simulink model "mini_projekt"  (R2020a)
settings: Solver=VariableStepAuto  StartTime=0.0  StopTime=10.0  MaxStep=0.1  RelTol=1e-3
values from neighbouring files (symbols this model uses):
  cp = 1000    [Skrypt.m]    (also in proj.m)
  Cv1 = cp*rop*V1    (= 90000)    [Skrypt.m]    (also in proj.m)
  Cv2 = cp*rop*V2    (= 90000)    [Skrypt.m]    (also in proj.m)
  dfp0 = 0*fpN    (= 0)    [Skrypt.m]    (also in proj.m)
  dTkz0 = 0    [Skrypt.m]    (also in proj.m)
  dTzew0 = 0    [Skrypt.m]    (also in proj.m)
  fp0 = fpN    (= 1.66666666667)    [Skrypt.m]    (also in proj.m)
  K0 = (qkN - Ks1*(Tw1N-TzewN))/(Tw1N-Tw2N)    (= 1600)    [Skrypt.m]    (also in proj.m)
  Ks1 = 0.6*qkN/(Tw1N-TzewN)    (= 300)    [Skrypt.m]    (also in proj.m)
  Ks2 = (K0*(Tw1N-Tw2N)+xpN*Tw1N-xpN*Tw2N)/(Tw2N-TzewN)    (= 514.285714286)    [Skrypt.m]    (also in proj.m)
  rop = 1.2    [Skrypt.m]    (also in proj.m)
  steptime = 50    [proj.m]
  Tkz0 = TkzN    (= 30)    [Skrypt.m]    (also in proj.m)
  Tw10 = (((xp0*Tkz1 + Ks1*Tzew0)*(K0+xp0+Ks2))+ Ks2*Tzew0*K0)/((xp0+Ks1+K0)*(K0+xp0+Ks2)-(K0^2+xp0*K0))    [Skrypt.m]    (also in proj.m)
  Tw20 = (Tw10*(K0+xp0) + Ks2*Tzew0)/(K0 + xp0 + Ks2)    (= 15)    [Skrypt.m]    (also in proj.m)
  Tzew0 = TzewN    (= -20)    [Skrypt.m]    (also in proj.m)
settings Model: Creator=swier  LastModifiedBy=pc

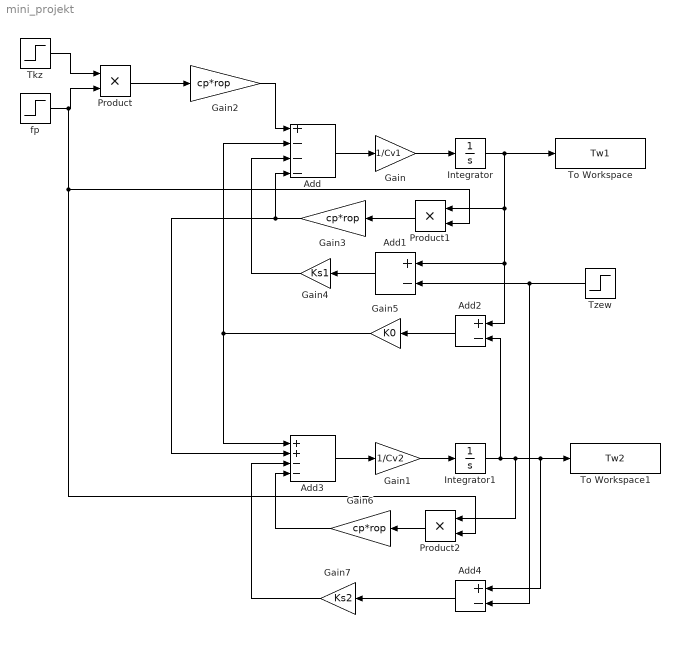
== system mini_projekt ==
  Add : Sum  Inputs=+---
  Add1 : Sum  Inputs=+-
  Add2 : Sum  Inputs=+-
  Add3 : Sum  Inputs=++--
  Add4 : Sum  Inputs=+-
  Gain : Gain  Gain=1/Cv1
  Gain1 : Gain  Gain=1/Cv2
  Gain2 : Gain  Gain=cp*rop
  Gain3 : Gain  Gain=cp*rop
  Gain4 : Gain  Gain=Ks1
  Gain5 : Gain  Gain=K0
  Gain6 : Gain  Gain=cp*rop
  Gain7 : Gain  Gain=Ks2
  Integrator : Integrator  InitialCondition=Tw10
  Integrator1 : Integrator  InitialCondition=Tw20
  Product : Product
  Product1 : Product
  Product2 : Product
  Tkz : Step  Time=steptime  Before=Tkz0  After=Tkz0+dTkz0  SampleTime=0
  To Workspace : ToWorkspace  VariableName=Tw1  SampleTime=-1
  To Workspace1 : ToWorkspace  VariableName=Tw2  SampleTime=-1
  Tzew : Step  Time=steptime  Before=Tzew0  After=Tzew0+dTzew0  SampleTime=0
  fp : Step  Time=steptime  Before=fp0  After=fp0+dfp0  SampleTime=0
  wires:
  Tkz/1 -> Product/1
  Add/1 -> Gain/1
  Gain/1 -> Integrator/1
  Gain1/1 -> Integrator1/1
  Integrator1/1 -> Add4/1, To Workspace1/1, Product2/1, Add2/2
  Integrator/1 -> Add2/1, Add1/1, Product1/1, To Workspace/1
  Gain3/1 -> Add/4, Add3/2
  Add1/1 -> Gain4/1
  Gain4/1 -> Add/3
  Add2/1 -> Gain5/1
  Gain5/1 -> Add3/1, Add/2
  Add3/1 -> Gain1/1
  Gain6/1 -> Add3/4
  Tzew/1 -> Add4/2, Add1/2
  Add4/1 -> Gain7/1
  Gain7/1 -> Add3/3
  Product/1 -> Gain2/1
  Product1/1 -> Gain3/1
  Product2/1 -> Gain6/1
  fp/1 -> Product2/2, Product1/2, Product/2
  Gain2/1 -> Add/1
